simulink model "EVX_Lap_Simulation 2"  (R2018b)
settings: Solver=FixedStepAuto  StartTime=0  StopTime=120  FixedStep=0.001  MaxStep=0.01  RelTol=1e-2
values from neighbouring files (symbols this model uses):
  velocity_dnew = velocity_d + 0.4 .* (velocity_dmax - velocity_d)    [Run_Sim(with_fmincon).m]
undefined symbols (not defined in the file or in its folder): dist, theta_d
libraries: simulink x1
(part 1 of 3)
settings Model: Creator=Foster  LastModifiedBy=Foster
settings SolverCC: AlgebraicLoopSolver=LineSearch
settings DebuggingCC: UnderSpecifiedDimensionMsg=warning
settings HardwareCC: ProdBitPerLong=64  ProdHWDeviceType=Intel->x86-64 (Mac OS X)

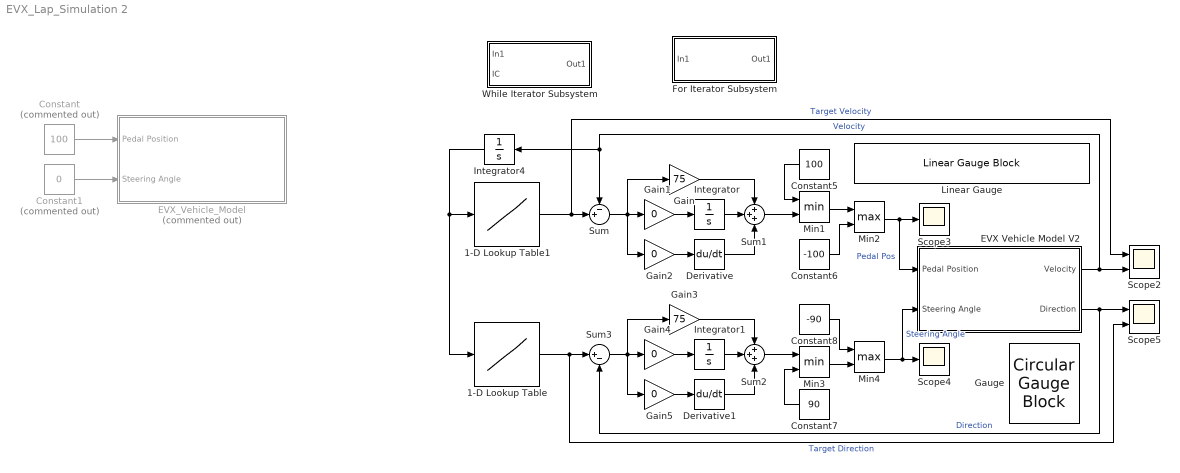
== system EVX_Lap_Simulation 2 ==
  1-D Lookup Table : Lookup_n-D  NumberOfTableDimensions=1  BreakpointsForDimension1=dist  Table=theta_d  ExtrapMethod=Clip  InternalRulePriority=Speed  RndMeth=Simplest  InputSameDT=on
  1-D Lookup Table1 : Lookup_n-D  NumberOfTableDimensions=1  BreakpointsForDimension1=dist  Table=velocity_dnew  ExtrapMethod=Clip  InternalRulePriority=Speed  RndMeth=Simplest  InputSameDT=on
  Constant : Constant  Commented=on  Value=100
  Constant1 : Constant  Commented=on  Value=0
  Constant5 : Constant  Value=100
  Constant6 : Constant  Value=-100
  Constant7 : Constant  Value=90
  Constant8 : Constant  Value=-90
  Derivative : Derivative
  Derivative1 : Derivative
  EVX Vehicle Model V2 : Subsystem
  EVX_Vehicle_Model : Subsystem  Commented=on
  For Iterator Subsystem : Subsystem  TreatAsAtomicUnit=on
  Gain : Gain  Gain=75
  Gain{1..2,4..5} (4 alike) : Gain  Gain=0
  Gain3 : Gain  Gain=75
  Gauge : CircularGaugeBlock  WebBlockId=1272  ScaleMin=-90  ScaleMax=90
  Integrator : Integrator
  Integrator1 : Integrator
  Integrator4 : Integrator
  Linear Gauge : LinearGaugeBlock  WebBlockId=1271  ScaleMin=-100
  Min1 : MinMax  Inputs=2
  Min2 : MinMax  Function=max  Inputs=2
  Min3 : MinMax  Inputs=2
  Min4 : MinMax  Function=max  Inputs=2
  Scope2 : Scope  NumInputPorts=2
  Scope3 : Scope
  Scope4 : Scope
  Scope5 : Scope  NumInputPorts=2
  Sum : Sum  Inputs=-+|
  Sum1 : Sum  Inputs=+++
  Sum2 : Sum  Inputs=+++
  Sum3 : Sum  Inputs=|+-
  While Iterator Subsystem : Subsystem  TreatAsAtomicUnit=on
  wires:
  Constant/1 -> EVX_Vehicle_Model/1(Pedal Position)
  Constant1/1 -> EVX_Vehicle_Model/2(Steering Angle)
  EVX Vehicle Model V2/1(Velocity) -> Scope2/2, Integrator4/1, Sum/1  "Velocity"
  Sum/1 -> Gain2/1, Gain/1, Gain1/1
  Integrator/1 -> Sum1/2
  Sum1/1 -> Min1/2
  Derivative/1 -> Sum1/3
  Gain/1 -> Sum1/1
  Gain1/1 -> Integrator/1
  Gain2/1 -> Derivative/1
  Constant5/1 -> Min1/1
  Derivative1/1 -> Sum2/3
  Gain5/1 -> Derivative1/1
  Gain3/1 -> Sum2/1
  Gain4/1 -> Integrator1/1
  Sum3/1 -> Gain5/1, Gain3/1, Gain4/1
  Integrator1/1 -> Sum2/2
  Min2/1 -> Scope3/1, EVX Vehicle Model V2/1(Pedal Position)  "Pedal Pos"
  Min1/1 -> Min2/1
  Constant6/1 -> Min2/2
  Min4/1 -> EVX Vehicle Model V2/2(Steering Angle), Scope4/1  "Steering Angle"
  Sum2/1 -> Min3/1
  Constant7/1 -> Min3/2
  Min3/1 -> Min4/2
  Constant8/1 -> Min4/1
  EVX Vehicle Model V2/2(Direction) -> Sum3/2, Scope5/1  "Direction"
  1-D Lookup Table/1 -> Scope5/2, Sum3/1  "Target Direction"
  1-D Lookup Table1/1 -> Scope2/1, Sum/2  "Target Velocity"
  Integrator4/1 -> 1-D Lookup Table1/1, 1-D Lookup Table/1

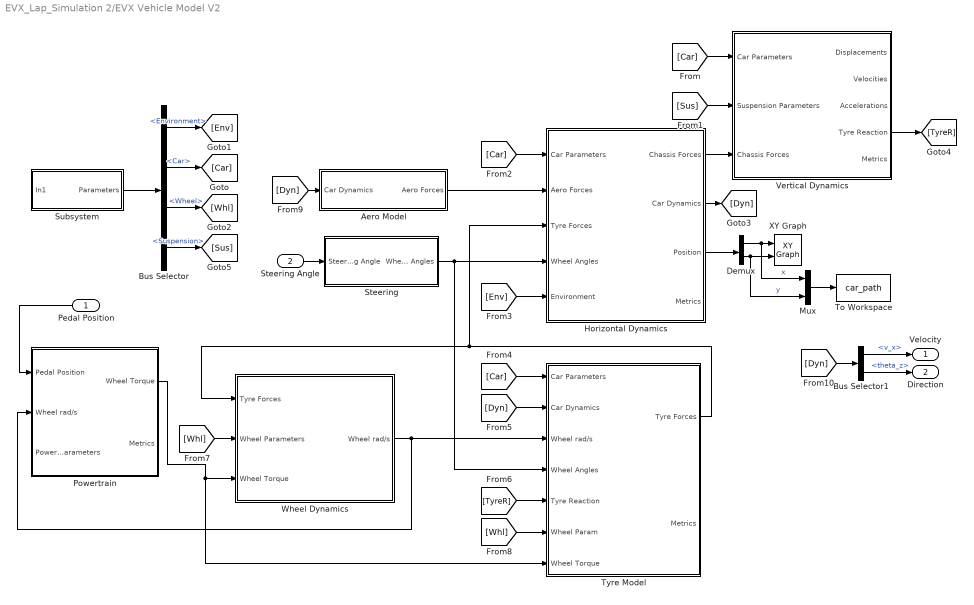
== system EVX_Lap_Simulation 2/EVX Vehicle Model V2 ==
  Pedal Position : Inport
  Steering Angle : Inport  Port=2
  Aero Model : Subsystem
  Bus Selector : BusSelector  OutputSignals=Environment,Car,Wheel,Suspension
  Bus Selector1 : BusSelector  OutputSignals=Velocities.v_x,Displacements.theta_z
  Demux : Demux  Outputs=2
  Horizontal Dynamics : Subsystem
  Mux : Mux  Inputs=2
  Powertrain : Subsystem
  Steering : Subsystem
  Subsystem : Subsystem
  To Workspace : ToWorkspace  VariableName=car_path  SaveFormat=Timeseries  SampleTime=-1
  Tyre Model : Subsystem
  Vertical Dynamics : Subsystem
  Wheel Dynamics : Subsystem
  XY Graph : simulink/Sinks/XY Graph  xmin=-400  xmax=100  ymin=-25  ymax=250  st=-1
  Velocity : Outport
  Direction : Outport  Port=2
  wires:
  [Car] -> Vertical Dynamics/1(Car Parameters)
  [Sus] -> Vertical Dynamics/2(Suspension Parameters)
  [Car] -> Horizontal Dynamics/1(Car Parameters)
  Horizontal Dynamics/3(Position) -> Demux/1
  Demux/1 -> Mux/1, XY Graph/1  "x"
  Demux/2 -> Mux/2, XY Graph/2  "y"
  Steering Angle/1 -> Steering/1(Steering Angle)
  Steering/1(Wheel Angles) -> Tyre Model/4(Wheel Angles), Horizontal Dynamics/4(Wheel Angles)
  [Env] -> Horizontal Dynamics/5(Environment)
  [Car] -> Tyre Model/1(Car Parameters)
  Horizontal Dynamics/2(Car Dynamics) -> [Dyn]
  [Dyn] -> Tyre Model/2(Car Dynamics)
  [TyreR] -> Tyre Model/5(Tyre Reaction)
  [Whl] -> Wheel Dynamics/2(Wheel Parameters)
  Pedal Position/1 -> Powertrain/1(Pedal Position)
  Powertrain/1(Wheel Torque) -> Tyre Model/7(Wheel Torque), Wheel Dynamics/3(Wheel Torque)
  [Whl] -> Tyre Model/6(Wheel Param)
  Subsystem/1(Parameters) -> Bus Selector/1
  Bus Selector/1 -> [Env]  "<Environment>"
  Bus Selector/2 -> [Car]  "<Car>"
  Bus Selector/3 -> [Whl]  "<Wheel>"
  Bus Selector/4 -> [Sus]  "<Suspension>"
  [Dyn] -> Aero Model/1(Car Dynamics)
  Aero Model/1(Aero Forces) -> Horizontal Dynamics/2(Aero Forces)
  Horizontal Dynamics/1(Chassis Forces) -> Vertical Dynamics/3(Chassis Forces)
  Vertical Dynamics/4(Tyre Reaction) -> [TyreR]
  Wheel Dynamics/1(Wheel rad/s) -> Powertrain/2(Wheel rad/s), Tyre Model/3(Wheel rad/s)
  Tyre Model/1(Tyre Forces) -> Wheel Dynamics/1(Tyre Forces), Horizontal Dynamics/3(Tyre Forces)
  [Dyn] -> Bus Selector1/1
  Bus Selector1/1 -> Velocity/1  "<v_x>"
  Bus Selector1/2 -> Direction/1  "<theta_z>"
  Mux/1 -> To Workspace/1

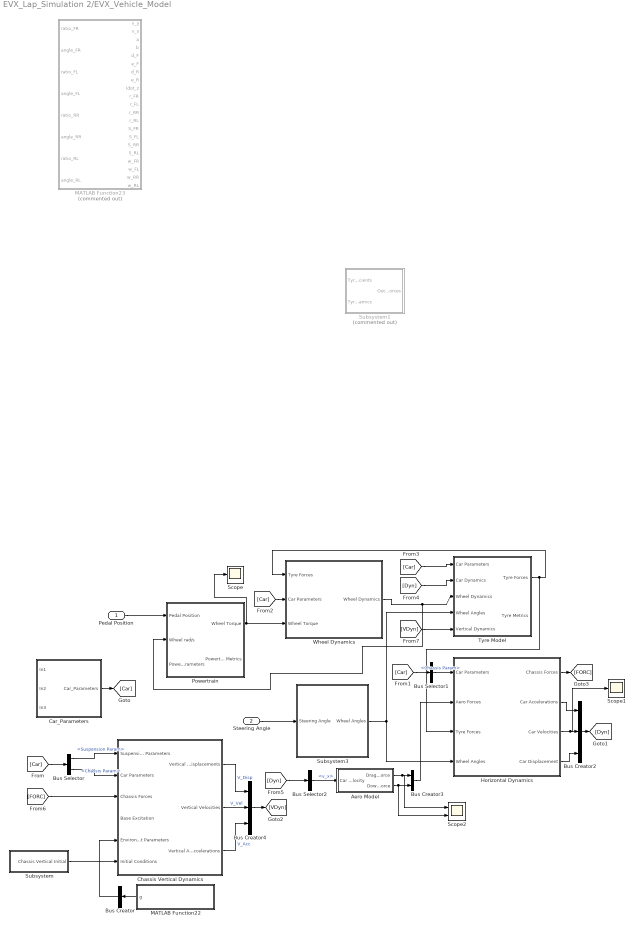
== system EVX_Lap_Simulation 2/EVX_Vehicle_Model ==
  Pedal Position : Inport
  Steering Angle : Inport  Port=2
  Aero Model : Subsystem
  Bus Creator : BusCreator  Inputs=1
  Bus Creator2 : BusCreator  Inputs=3
  Bus Creator3 : BusCreator  Inputs=2
  Bus Creator4 : BusCreator  Inputs=3
  Bus Selector : BusSelector  OutputSignals=Suspension Param,Chassis Param
  Bus Selector1 : BusSelector  OutputSignals=Chassis Param
  Bus Selector2 : BusSelector  OutputSignals=Car Velocities.v_x
  Car_Parameters : Subsystem
  Chassis Vertical Dynamics : Subsystem
  Horizontal Dynamics : Subsystem
  MATLAB Function22 : MATLAB Function  TreatAsAtomicUnit=on
  MATLAB Function23 : MATLAB Function  Commented=on  TreatAsAtomicUnit=on
  Powertrain : Subsystem
  Scope : Scope
  Scope1 : Scope
  Scope2 : Scope  NumInputPorts=2
  Subsystem : Subsystem
  Subsystem1 : Subsystem  Commented=on
  Subsystem3 : Subsystem
  Tyre Model : Subsystem
  Wheel Dynamics : Subsystem
  wires:
  Subsystem/1(Chassis Vertical Initial) -> Chassis Vertical Dynamics/6(Initial Conditions)
  MATLAB Function22/1(g) -> Bus Creator/1
  Bus Selector/1 -> Chassis Vertical Dynamics/1(Suspension Parameters)  "<Suspension Param>"
  Bus Selector1/1 -> Horizontal Dynamics/1(Car Parameters)  "<Chassis Param>"
  [Car] -> Bus Selector/1
  Bus Selector/2 -> Chassis Vertical Dynamics/2(Car Parameters)  "<Chassis Param>"
  Car_Parameters/1(Car_Parameters) -> [Car]
  [Car] -> Bus Selector1/1
  Bus Creator/1 -> Chassis Vertical Dynamics/5(Environment Parameters)
  Pedal Position/1 -> Powertrain/1(Pedal Position)
  Powertrain/1(Wheel Torque) -> Wheel Dynamics/3(Wheel Torque), Scope/1
  [Car] -> Wheel Dynamics/2(Car Parameters)
  [Car] -> Tyre Model/1(Car Parameters)
  Tyre Model/1(Tyre Forces) -> Horizontal Dynamics/3(Tyre Forces), Wheel Dynamics/1(Tyre Forces)
  Horizontal Dynamics/3(Car Velocities) -> Scope1/1, Bus Creator2/2
  Horizontal Dynamics/4(Car Displacement) -> Bus Creator2/3
  Horizontal Dynamics/2(Car Accelerations) -> Bus Creator2/1
  Bus Creator2/1 -> [Dyn]
  [Dyn] -> Tyre Model/2(Car Dynamics)
  Wheel Dynamics/1(Wheel Dynamics) -> Tyre Model/3(Wheel Dynamics), Powertrain/2(Wheel rad/s)
  Subsystem3/1(Wheel Angles) -> Tyre Model/4(Wheel Angles), Horizontal Dynamics/4(Wheel Angles)
  Steering Angle/1 -> Subsystem3/1(Steering Angle)
  [Dyn] -> Bus Selector2/1
  Bus Selector2/1 -> Aero Model/1(Car Velocity)  "<v_x>"
  Aero Model/1(Drag Force) -> Scope2/1, Bus Creator3/1
  Aero Model/2(Down Force) -> Scope2/2, Bus Creator3/2
  Bus Creator3/1 -> Horizontal Dynamics/2(Aero Forces)
  Chassis Vertical Dynamics/2(Vertical Velocities) -> Bus Creator4/2  "V_Vel"
  Chassis Vertical Dynamics/1(Vertical Displacements) -> Bus Creator4/1  "V_Disp"
  Chassis Vertical Dynamics/3(Vertical Accelerations) -> Bus Creator4/3  "V_Acc"
  Bus Creator4/1 -> [VDyn]
  Horizontal Dynamics/1(Chassis Forces) -> [FORC]
  [FORC] -> Chassis Vertical Dynamics/3(Chassis Forces)
  [VDyn] -> Tyre Model/5(Vertical Dynamics)

== system EVX_Lap_Simulation 2/For Iterator Subsystem ==
  In1 : Inport
  For Iterator : ForIterator
  Out1 : Outport
  wires:
  In1/1 -> Out1/1

== system EVX_Lap_Simulation 2/While Iterator Subsystem ==
  In1 : Inport
  IC : Inport  Port=2
  While Iterator : WhileIterator  ShowIterationPort=on
  Out1 : Outport
  wires:
  IC/1 -> While Iterator/2
  In1/1 -> Out1/1

== system EVX_Lap_Simulation 2/EVX Vehicle Model V2/Aero Model ==
  Car Dynamics : Inport
  Bus Creator : BusCreator  Inputs=2
  Bus Creator1 : BusCreator  Inputs=2
  Bus Creator2 : BusCreator  Inputs=2
  Bus Selector : BusSelector  OutputSignals=Velocities.v_x
  Forces : MATLAB Function  TreatAsAtomicUnit=on
  Interpreted MATLAB Function : MATLABFcn  MATLABFcn=Vel_update  Output1D=off
  Position : MATLAB Function  TreatAsAtomicUnit=on
  Aero Forces : Outport
  wires:
  Car Dynamics/1 -> Bus Selector/1
  Bus Selector/1 -> Forces/1(v_x), Position/1(v_x)  "<v_x>"
  Forces/1(F_L) -> Bus Creator/1
  Forces/2(F_D) -> Bus Creator/2
  Position/1(L) -> Bus Creator1/1
  Position/2(D) -> Bus Creator1/2
  Bus Creator/1 -> Bus Creator2/1  "Forces"
  Bus Creator1/1 -> Bus Creator2/2  "Position"
  Bus Creator2/1 -> Aero Forces/1

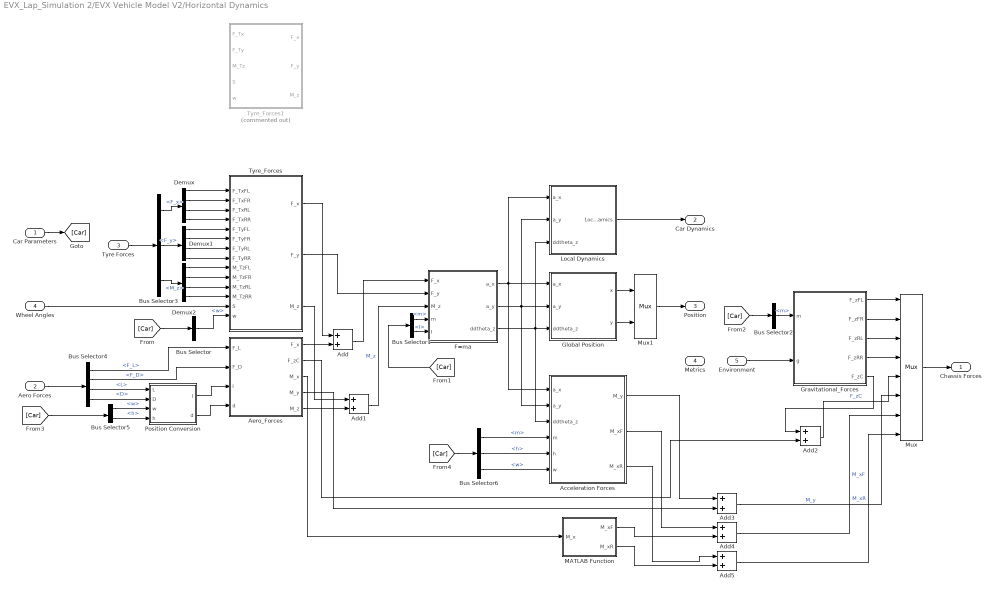
== system EVX_Lap_Simulation 2/EVX Vehicle Model V2/Horizontal Dynamics ==
  Car Parameters : Inport
  Aero Forces : Inport  Port=2
  Tyre Forces : Inport  Port=3
  Wheel Angles : Inport  Port=4
  Environment : Inport  Port=5
  Acceleration Forces : MATLAB Function  TreatAsAtomicUnit=on
  Add{,1..5} (6 alike) : Sum
  Aero_Forces : MATLAB Function  TreatAsAtomicUnit=on
  Bus Selector : BusSelector  OutputSignals=w
  Bus Selector1 : BusSelector  OutputSignals=m,I
  Bus Selector2 : BusSelector  OutputSignals=m
  Bus Selector3 : BusSelector  OutputSignals=F_x,F_y,M_z
  Bus Selector4 : BusSelector  OutputSignals=Forces.F_L,Forces.F_D,Position.L,Position.D
  Bus Selector5 : BusSelector  OutputSignals=w,h
  Bus Selector6 : BusSelector  OutputSignals=m,h,w
  Demux : Demux
  Demux1 : Demux
  Demux2 : Demux
  F=ma : MATLAB Function  TreatAsAtomicUnit=on
  Global Position : Subsystem
  Gravitational_Forces : MATLAB Function  TreatAsAtomicUnit=on
  Local Dynamics : Subsystem
  MATLAB Function : MATLAB Function  TreatAsAtomicUnit=on
  Mux : Mux  Inputs=8
      settings: DisplayOption=signals
  Mux1 : Mux  Inputs=2
      settings: DisplayOption=signals
  Position Conversion : MATLAB Function  TreatAsAtomicUnit=on
  Tyre_Forces : MATLAB Function  TreatAsAtomicUnit=on
  Tyre_Forces1 : MATLAB Function  Commented=on  TreatAsAtomicUnit=on
  Chassis Forces : Outport
  Car Dynamics : Outport  Port=2
  Position : Outport  Port=3
  Metrics : Outport  Port=4
  wires:
  Car Parameters/1 -> [Car]
  [Car] -> Bus Selector/1
  Bus Selector/1 -> Tyre_Forces/14(w)  "<w>"
  Add2/1 -> Mux/5  "F_zC"
  Add1/1 -> F=ma/3(M_z)  "M_z"
  Add/1 -> F=ma/1(F_x)
  [Car] -> Bus Selector1/1
  Bus Selector1/1 -> F=ma/4(m)  "<m>"
  Bus Selector1/2 -> F=ma/5(I)  "<I>"
  F=ma/1(a_x) -> Local Dynamics/1(a_x), Global Position/1(a_x), Acceleration Forces/1(a_x)
  F=ma/2(a_y) -> Local Dynamics/2(a_y), Global Position/2(a_y), Acceleration Forces/2(a_y)
  F=ma/3(ddtheta_z) -> Local Dynamics/3(ddtheta_z), Global Position/3(ddtheta_z), Acceleration Forces/3(ddtheta_z)
  Bus Selector2/1 -> Gravitational_Forces/1(m)  "<m>"
  [Car] -> Bus Selector2/1
  Global Position/1(x) -> Mux1/1
  Global Position/2(y) -> Mux1/2
  Mux1/1 -> Position/1
  Environment/1 -> Gravitational_Forces/2(g)
  Local Dynamics/1(Local Dynamics) -> Car Dynamics/1
  Wheel Angles/1 -> Tyre_Forces/13(S)
  Aero Forces/1 -> Bus Selector4/1
  Bus Selector4/1 -> Aero_Forces/1(F_L)  "<F_L>"
  Bus Selector4/2 -> Aero_Forces/2(F_D)  "<F_D>"
  Bus Selector4/3 -> Position Conversion/1(L)  "<L>"
  Bus Selector4/4 -> Position Conversion/2(D)  "<D>"
  Position Conversion/1(l) -> Aero_Forces/3(l)
  Position Conversion/2(d) -> Aero_Forces/4(d)
  [Car] -> Bus Selector5/1
  Bus Selector5/1 -> Position Conversion/3(w)  "<w>"
  Bus Selector5/2 -> Position Conversion/4(h)  "<h>"
  Mux/1 -> Chassis Forces/1
  [Car] -> Bus Selector6/1
  Bus Selector6/1 -> Acceleration Forces/4(m)  "<m>"
  Bus Selector6/2 -> Acceleration Forces/5(h)  "<h>"
  Bus Selector6/3 -> Acceleration Forces/6(w)  "<w>"
  Gravitational_Forces/5(F_zC) -> Add2/1
  Gravitational_Forces/4(F_zRR) -> Mux/4
  Gravitational_Forces/3(F_zRL) -> Mux/3
  Gravitational_Forces/2(F_zFR) -> Mux/2
  Gravitational_Forces/1(F_zFL) -> Mux/1
  Aero_Forces/2(F_zC) -> Add2/2
  Aero_Forces/5(M_z) -> Add1/2
  Tyre_Forces/3(M_z) -> Add1/1
  Aero_Forces/1(F_x) -> Add/2
  Tyre_Forces/1(F_x) -> Add/1
  Tyre_Forces/2(F_y) -> F=ma/2(F_y)
  Aero_Forces/3(M_x) -> MATLAB Function/1(M_x)
  Aero_Forces/4(M_y) -> Add3/2
  Acceleration Forces/1(M_y) -> Add3/1
  Add3/1 -> Mux/6  "M_y"
  Acceleration Forces/2(M_xF) -> Add4/1
  MATLAB Function/1(M_xF) -> Add4/2
  Acceleration Forces/3(M_xR) -> Add5/1
  MATLAB Function/2(M_xR) -> Add5/2
  Add4/1 -> Mux/7  "M_xF"
  Add5/1 -> Mux/8  "M_xR"
  Tyre Forces/1 -> Bus Selector3/1
  Bus Selector3/1 -> Demux/1  "<F_x>"
  Bus Selector3/2 -> Demux1/1  "<F_y>"
  Bus Selector3/3 -> Demux2/1  "<M_z>"
  Demux/1 -> Tyre_Forces/1(F_TxFL)
  Demux/2 -> Tyre_Forces/2(F_TxFR)
  Demux/3 -> Tyre_Forces/3(F_TxRL)
  Demux/4 -> Tyre_Forces/4(F_TxRR)
  Demux1/1 -> Tyre_Forces/5(F_TyFL)
  Demux1/2 -> Tyre_Forces/6(F_TyFR)
  Demux1/3 -> Tyre_Forces/7(F_TyRL)
  Demux1/4 -> Tyre_Forces/8(F_TyRR)
  Demux2/1 -> Tyre_Forces/9(M_TzFL)
  Demux2/2 -> Tyre_Forces/10(M_TzFR)
  Demux2/3 -> Tyre_Forces/11(M_TzRL)
  Demux2/4 -> Tyre_Forces/12(M_TzRR)

== system EVX_Lap_Simulation 2/EVX Vehicle Model V2/Powertrain ==
  Pedal Position : Inport
  Wheel rad/s : Inport  Port=2
  Powertrain Parameters : Inport  Port=3
  Brake Function : MATLAB Function  TreatAsAtomicUnit=on
  Constant : Constant  Value=3
  Constant1 : Constant
  Constant2 : Constant
  Demux1 : Demux
  Demux2 : Demux
  Motor Fucntion : MATLAB Function  TreatAsAtomicUnit=on
  Mux : Mux
      settings: DisplayOption=signals
  Reverse Transmission Function : MATLAB Function  TreatAsAtomicUnit=on
  Scope1 : Scope  NumInputPorts=4
  Scope2 : Scope  NumInputPorts=4
  Switch : Switch
  Transmission Function : MATLAB Function  TreatAsAtomicUnit=on
  Wheel Torque : Outport
  Metrics : Outport  Port=2
  wires:
  Constant/1 -> Transmission Function/1(Ratio), Reverse Transmission Function/1(Ratio)
  Constant1/1 -> Transmission Function/3(Splits)
  Reverse Transmission Function/1(Motor_Speed) -> Motor Fucntion/2(Motor_Speed)
  Mux/1 -> Switch/1
  Motor Fucntion/1(Torque) -> Transmission Function/2(Motor_Torque)
  Constant2/1 -> Motor Fucntion/3(Direction)
  Transmission Function/1(T_FL) -> Mux/1
  Transmission Function/2(T_FR) -> Mux/2
  Transmission Function/3(T_RL) -> Mux/3
  Transmission Function/4(T_RR) -> Mux/4
  Wheel rad/s/1 -> Demux2/1, Brake Function/1(v_wx), Reverse Transmission Function/2(dwheel)
  Demux1/4 -> Scope2/4  "T_RR"
  Demux1/3 -> Scope2/3  "T_RL"
  Demux1/1 -> Scope2/1  "T_FL"
  Demux1/2 -> Scope2/2  "T_FR"
  Pedal Position/1 -> Switch/2, Brake Function/2(Pedal), Motor Fucntion/1(Pedal)
  Switch/1 -> Demux1/1, Wheel Torque/1
  Brake Function/1(Torque) -> Switch/3
  Demux2/2 -> Scope1/2  "v_xwFR"
  Demux2/1 -> Scope1/1  "v_xwFL"
  Demux2/4 -> Scope1/4  "v_xwRR"
  Demux2/3 -> Scope1/3  "v_xwRL"

== system EVX_Lap_Simulation 2/EVX Vehicle Model V2/Steering ==
  Steering Angle : Inport
  Constant : Constant  Value=2
  Constant1 : Constant  Value=1.5
  Front/Rear Split : MATLAB Function  TreatAsAtomicUnit=on
  MATLAB Function : MATLAB Function  TreatAsAtomicUnit=on
  MATLAB Function1 : MATLAB Function  TreatAsAtomicUnit=on
  Mux : Mux
  Wheel Angles : Outport
  wires:
  Steering Angle/1 -> Front/Rear Split/1(Angle)
  Front/Rear Split/1(Steering_F) -> MATLAB Function/1(Steering_F)
  Front/Rear Split/2(Steering_R) -> MATLAB Function1/1(Steering_R)
  Constant/1 -> MATLAB Function/2(Ratio)
  Constant1/1 -> MATLAB Function1/2(Ratio)
  Mux/1 -> Wheel Angles/1
  MATLAB Function/1(S_FL) -> Mux/1
  MATLAB Function/2(S_FR) -> Mux/2
  MATLAB Function1/1(S_RL) -> Mux/3
  MATLAB Function1/2(S_RR) -> Mux/4

== system EVX_Lap_Simulation 2/EVX Vehicle Model V2/Subsystem ==
  In1 : Inport
  Bus Creator : BusCreator  Inputs=6
  Bus Creator1 : BusCreator  Inputs=6
  Bus Creator2 : BusCreator  Inputs=2
  Bus Creator3 : BusCreator  Inputs=1
  Bus Creator4 : BusCreator  Inputs=4
  Car Parameters : MATLAB Function  TreatAsAtomicUnit=on
  Environment Parameters : MATLAB Function  TreatAsAtomicUnit=on
  Suspension Parameters : MATLAB Function  TreatAsAtomicUnit=on
  Wheel Parameters : MATLAB Function  TreatAsAtomicUnit=on
  Parameters : Outport
  wires:
  Suspension Parameters/4(ct) -> Bus Creator/4
  Suspension Parameters/5(cs) -> Bus Creator/5
  Suspension Parameters/1(kt) -> Bus Creator/1
  Suspension Parameters/3(kr) -> Bus Creator/3
  Bus Creator/1 -> Bus Creator4/4  "Suspension"
  Car Parameters/1(w) -> Bus Creator1/1
  Bus Creator2/1 -> Bus Creator4/3  "Wheel"
  Bus Creator1/1 -> Bus Creator4/2  "Car"
  Suspension Parameters/2(ks) -> Bus Creator/2
  Car Parameters/5(cc) -> Bus Creator1/5
  Wheel Parameters/2(I) -> Bus Creator2/2
  Car Parameters/3(I) -> Bus Creator1/3
  Suspension Parameters/6(cr) -> Bus Creator/6
  Car Parameters/2(m) -> Bus Creator1/2
  Car Parameters/4(kc) -> Bus Creator1/4
  Wheel Parameters/1(r) -> Bus Creator2/1
  Environment Parameters/1(g) -> Bus Creator3/1
  Bus Creator3/1 -> Bus Creator4/1  "Environment"
  Bus Creator4/1 -> Parameters/1
  Car Parameters/6(h) -> Bus Creator1/6

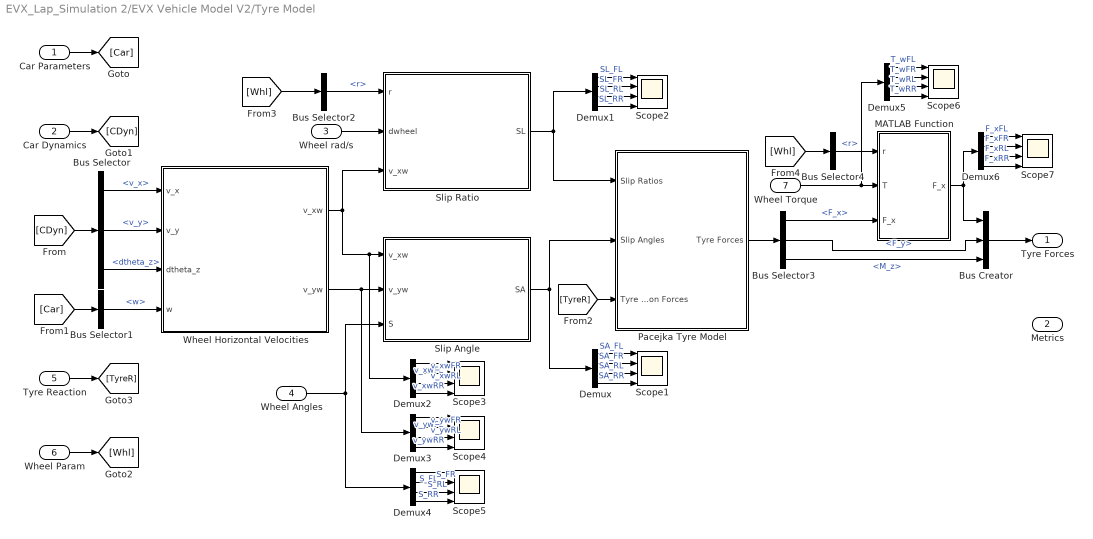
== system EVX_Lap_Simulation 2/EVX Vehicle Model V2/Tyre Model ==
  Car Parameters : Inport
  Car Dynamics : Inport  Port=2
  Wheel rad/s : Inport  Port=3
  Wheel Angles : Inport  Port=4
  Tyre Reaction : Inport  Port=5
  Wheel Param : Inport  Port=6
  Wheel Torque : Inport  Port=7
  Bus Creator : BusCreator  Inputs=3
  Bus Selector : BusSelector  OutputSignals=Velocities.v_x,Velocities.v_y,Velocities.dtheta_z
  Bus Selector1 : BusSelector  OutputSignals=w
  Bus Selector2 : BusSelector  OutputSignals=r
  Bus Selector3 : BusSelector  OutputSignals=F_x,F_y,M_z
  Bus Selector4 : BusSelector  OutputSignals=r
  Demux{,1..6} (7 alike) : Demux
  MATLAB Function : MATLAB Function  TreatAsAtomicUnit=on
  Pacejka Tyre Model : Subsystem
  Scope{1..7} (7 alike) : Scope  NumInputPorts=4
  Slip Angle : MATLAB Function  TreatAsAtomicUnit=on
  Slip Ratio : MATLAB Function  TreatAsAtomicUnit=on
  Wheel Horizontal Velocities : MATLAB Function  TreatAsAtomicUnit=on
  Tyre Forces : Outport
  Metrics : Outport  Port=2
  wires:
  Car Parameters/1 -> [Car]
  Car Dynamics/1 -> [CDyn]
  Wheel rad/s/1 -> Slip Ratio/2(dwheel)
  [CDyn] -> Bus Selector/1
  Bus Selector/3 -> Wheel Horizontal Velocities/3(dtheta_z)  "<dtheta_z>"
  [Car] -> Bus Selector1/1
  Bus Selector1/1 -> Wheel Horizontal Velocities/4(w)  "<w>"
  Tyre Reaction/1 -> [TyreR]
  [TyreR] -> Pacejka Tyre Model/3(Tyre Reaction Forces)
  Slip Angle/1(SA) -> Demux/1, Pacejka Tyre Model/2(Slip Angles)
  Slip Ratio/1(SL) -> Demux1/1, Pacejka Tyre Model/1(Slip Ratios)
  Bus Selector/1 -> Wheel Horizontal Velocities/1(v_x)  "<v_x>"
  Bus Selector/2 -> Wheel Horizontal Velocities/2(v_y)  "<v_y>"
  Wheel Horizontal Velocities/1(v_xw) -> Slip Ratio/3(v_xw), Demux2/1, Slip Angle/1(v_xw)
  Wheel Horizontal Velocities/2(v_yw) -> Demux3/1, Slip Angle/2(v_yw)
  Wheel Angles/1 -> Slip Angle/3(S), Demux4/1
  Wheel Param/1 -> [Whl]
  [Whl] -> Bus Selector2/1
  Bus Selector2/1 -> Slip Ratio/1(r)  "<r>"
  Demux/1 -> Scope1/1  "SA_FL"
  Demux/2 -> Scope1/2  "SA_FR"
  Demux/3 -> Scope1/3  "SA_RL"
  Demux/4 -> Scope1/4  "SA_RR"
  Demux1/1 -> Scope2/1  "SL_FL"
  Demux1/2 -> Scope2/2  "SL_FR"
  Demux1/3 -> Scope2/3  "SL_RL"
  Demux1/4 -> Scope2/4  "SL_RR"
  Pacejka Tyre Model/1(Tyre Forces) -> Bus Selector3/1
  [Whl] -> Bus Selector4/1
  Bus Selector4/1 -> MATLAB Function/1(r)  "<r>"
  Wheel Torque/1 -> MATLAB Function/2(T), Demux5/1
  Bus Selector3/1 -> MATLAB Function/3("F_x ")  "<F_x>"
  MATLAB Function/1(F_x) -> Bus Creator/1, Demux6/1
  Bus Selector3/2 -> Bus Creator/2  "<F_y>"
  Bus Selector3/3 -> Bus Creator/3  "<M_z>"
  Bus Creator/1 -> Tyre Forces/1
  Demux2/4 -> Scope3/4  "v_xwRR"
  Demux2/1 -> Scope3/1  "v_xwFL"
  Demux2/3 -> Scope3/3  "v_xwRL"
  Demux2/2 -> Scope3/2  "v_xwFR"
  Demux3/4 -> Scope4/4  "v_ywRR"
  Demux3/1 -> Scope4/1  "v_ywFL"
  Demux3/3 -> Scope4/3  "v_ywRL"
  Demux3/2 -> Scope4/2  "v_ywFR"
  Demux4/4 -> Scope5/4  "S_RR"
  Demux4/1 -> Scope5/1  "S_FL"
  Demux4/3 -> Scope5/3  "S_RL"
  Demux4/2 -> Scope5/2  "S_FR"
  Demux5/3 -> Scope6/3  "T_wRL"
  Demux5/4 -> Scope6/4  "T_wRR"
  Demux5/1 -> Scope6/1  "T_wFL"
  Demux5/2 -> Scope6/2  "T_wFR"
  Demux6/3 -> Scope7/3  "F_xRL"
  Demux6/4 -> Scope7/4  "F_xRR"
  Demux6/1 -> Scope7/1  "F_xFL"
  Demux6/2 -> Scope7/2  "F_xFR"

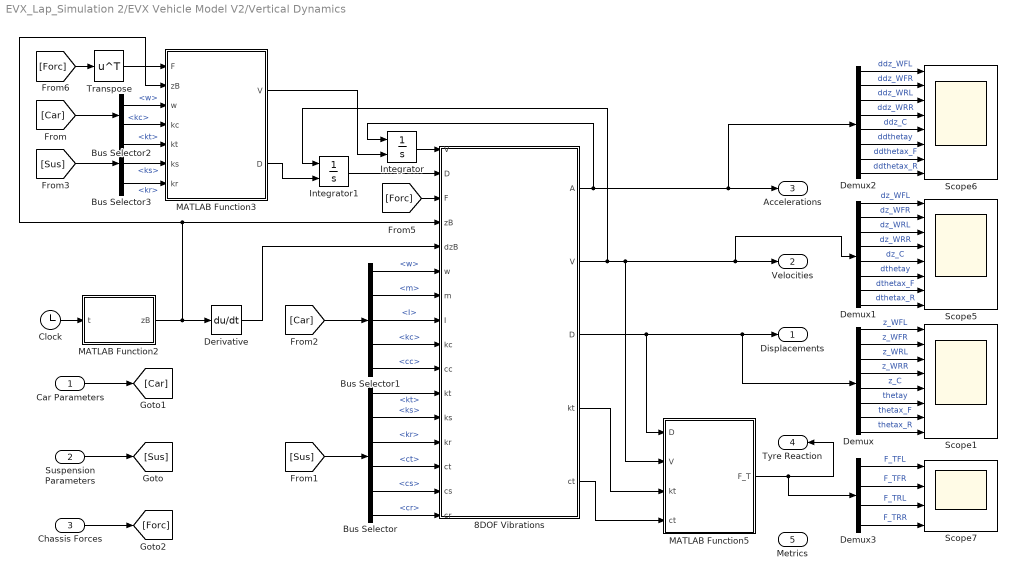
== system EVX_Lap_Simulation 2/EVX Vehicle Model V2/Vertical Dynamics ==
  Car Parameters : Inport
  Suspension Parameters : Inport  Port=2
  Chassis Forces : Inport  Port=3
  8DOF Vibrations : MATLAB Function  TreatAsAtomicUnit=on
  Bus Selector : BusSelector  OutputSignals=kt,ks,kr,ct,cs,cr
  Bus Selector1 : BusSelector  OutputSignals=w,m,I,kc,cc
  Bus Selector2 : BusSelector  OutputSignals=w,kc
  Bus Selector3 : BusSelector  OutputSignals=kt,ks,kr
  Clock : Clock
  Demux : Demux  Outputs=8
  Demux1 : Demux  Outputs=8
  Demux2 : Demux  Outputs=8
  Demux3 : Demux
  Derivative : Derivative
  Integrator : Integrator  InitialConditionSource=external
  Integrator1 : Integrator  InitialConditionSource=external
  MATLAB Function2 : MATLAB Function  TreatAsAtomicUnit=on
  MATLAB Function3 : MATLAB Function  TreatAsAtomicUnit=on
  MATLAB Function5 : MATLAB Function  TreatAsAtomicUnit=on
  Scope1 : Scope  NumInputPorts=8
  Scope5 : Scope  NumInputPorts=8
  Scope6 : Scope  NumInputPorts=8
  Scope7 : Scope  NumInputPorts=4
  Transpose : Math  Operator=transpose  SaturateOnIntegerOverflow=on
  Displacements : Outport
  Velocities : Outport  Port=2
  Accelerations : Outport  Port=3
  Tyre Reaction : Outport  Port=4
  Metrics : Outport  Port=5
  wires:
  Demux/1 -> Scope1/1  "z_WFL"
  Demux/2 -> Scope1/2  "z_WFR"
  Demux/3 -> Scope1/3  "z_WRL"
  Demux/4 -> Scope1/4  "z_WRR"
  Demux/5 -> Scope1/5  "z_C"
  Demux/6 -> Scope1/6  "thetay"
  Demux/7 -> Scope1/7  "thetax_F"
  Demux/8 -> Scope1/8  "thetax_R"
  8DOF Vibrations/3(D) -> Displacements/1, Demux/1, MATLAB Function5/1(D)
  Demux1/1 -> Scope5/1  "dz_WFL"
  Demux1/3 -> Scope5/3  "dz_WRL"
  Demux1/2 -> Scope5/2  "dz_WFR"
  Demux1/4 -> Scope5/4  "dz_WRR"
  Demux1/8 -> Scope5/8  "dthetax_R"
  Demux1/6 -> Scope5/6  "dthetay"
  Demux1/5 -> Scope5/5  "dz_C"
  Demux1/7 -> Scope5/7  "dthetax_F"
  8DOF Vibrations/2(V) -> Velocities/1, Demux1/1, MATLAB Function5/2(V), Integrator1/1
  Demux2/1 -> Scope6/1  "ddz_WFL"
  Demux2/3 -> Scope6/3  "ddz_WRL"
  Demux2/2 -> Scope6/2  "ddz_WFR"
  Demux2/4 -> Scope6/4  "ddz_WRR"
  Demux2/8 -> Scope6/8  "ddthetax_R"
  Demux2/6 -> Scope6/6  "ddthetay"
  Demux2/5 -> Scope6/5  "ddz_C"
  Demux2/7 -> Scope6/7  "ddthetax_F"
  8DOF Vibrations/1(A) -> Integrator/1, Accelerations/1, Demux2/1
  Demux3/1 -> Scope7/1  "F_TFL"
  Demux3/3 -> Scope7/3  "F_TRL"
  Demux3/2 -> Scope7/2  "F_TFR"
  Demux3/4 -> Scope7/4  "F_TRR"
  8DOF Vibrations/4(kt) -> MATLAB Function5/3(kt)
  8DOF Vibrations/5(ct) -> MATLAB Function5/4(ct)
  MATLAB Function2/1(zB) -> 8DOF Vibrations/4(zB), MATLAB Function3/2(zB), Derivative/1
  Derivative/1 -> 8DOF Vibrations/5(dzB)
  Integrator1/1 -> 8DOF Vibrations/2("D ")
  Integrator/1 -> 8DOF Vibrations/1("V ")
  Clock/1 -> MATLAB Function2/1(t)
  Suspension Parameters/1 -> [Sus]
  Car Parameters/1 -> [Car]
  [Sus] -> Bus Selector/1
  Bus Selector/1 -> 8DOF Vibrations/11("kt ")  "<kt>"
  Bus Selector/2 -> 8DOF Vibrations/12(ks)  "<ks>"
  Bus Selector/3 -> 8DOF Vibrations/13(kr)  "<kr>"
  Bus Selector/4 -> 8DOF Vibrations/14("ct ")  "<ct>"
  Bus Selector/5 -> 8DOF Vibrations/15(cs)  "<cs>"
  Bus Selector/6 -> 8DOF Vibrations/16(cr)  "<cr>"
  [Car] -> Bus Selector1/1
  Bus Selector1/1 -> 8DOF Vibrations/6(w)  "<w>"
  Bus Selector1/2 -> 8DOF Vibrations/7(m)  "<m>"
  Bus Selector1/4 -> 8DOF Vibrations/9(kc)  "<kc>"
  Bus Selector1/5 -> 8DOF Vibrations/10(cc)  "<cc>"
  [Car] -> Bus Selector2/1
  Bus Selector2/1 -> MATLAB Function3/3(w)  "<w>"
  Bus Selector2/2 -> MATLAB Function3/4(kc)  "<kc>"
  [Sus] -> Bus Selector3/1
  Bus Selector3/1 -> MATLAB Function3/5(kt)  "<kt>"
  Bus Selector3/2 -> MATLAB Function3/6(ks)  "<ks>"
  Bus Selector3/3 -> MATLAB Function3/7(kr)  "<kr>"
  MATLAB Function5/1(F_T) -> Demux3/1, Tyre Reaction/1
  MATLAB Function3/1(V) -> Integrator/2
  MATLAB Function3/2(D) -> Integrator1/2
  Bus Selector1/3 -> 8DOF Vibrations/8(I)  "<I>"
  Chassis Forces/1 -> [Forc]
  [Forc] -> 8DOF Vibrations/3(F)
  [Forc] -> Transpose/1
  Transpose/1 -> MATLAB Function3/1(F)

== system EVX_Lap_Simulation 2/EVX Vehicle Model V2/Wheel Dynamics ==
  Tyre Forces : Inport
  Wheel Parameters : Inport  Port=2
  Wheel Torque : Inport  Port=3
  Bus Selector : BusSelector  OutputSignals=F_x
  Bus Selector1 : BusSelector  OutputSignals=I,r
  Integrator : Integrator
  Scope{,1..3} (4 alike) : Scope
  Scope4 : Scope  NumInputPorts=2
  Wheel Acceleration : MATLAB Function  TreatAsAtomicUnit=on
  Wheel rad/s : Outport
  wires:
  Wheel Acceleration/1(ddwheel) -> Scope4/1, Integrator/1
  Wheel Parameters/1 -> Bus Selector1/1
  Bus Selector1/1 -> Scope/1, Wheel Acceleration/3(I)  "<I>"
  Bus Selector1/2 -> Scope3/1, Wheel Acceleration/4(r)  "<r>"
  Tyre Forces/1 -> Bus Selector/1
  Bus Selector/1 -> Scope2/1, Wheel Acceleration/1(F_x)  "<F_x>"
  Wheel Torque/1 -> Scope1/1, Wheel Acceleration/2(T)
  Integrator/1 -> Scope4/2, Wheel rad/s/1

== system EVX_Lap_Simulation 2/EVX_Vehicle_Model/Aero Model ==
  Car Velocity : Inport
  MATLAB Function : MATLAB Function  TreatAsAtomicUnit=on
  MATLAB Function1 : MATLAB Function  TreatAsAtomicUnit=on
  Drag Force : Outport
  Down Force : Outport  Port=2
  wires:
  MATLAB Function1/1(F_z) -> Down Force/1
  MATLAB Function/1(F_d) -> Drag Force/1
  Car Velocity/1 -> MATLAB Function1/1(v_x), MATLAB Function/1(v_x)

== system EVX_Lap_Simulation 2/EVX_Vehicle_Model/Car_Parameters ==
  In1 : Inport
  In2 : Inport  Port=2
  In3 : Inport  Port=3
  Bus Creator : BusCreator  Inputs=23
  Bus Creator1 : BusCreator  Inputs=4
  Bus Creator2 : BusCreator  Inputs=8
  Bus Creator6 : BusCreator  Inputs=59
  Bus Creator7 : BusCreator  Inputs=30
  MATLAB Function : MATLAB Function  TreatAsAtomicUnit=on
  MATLAB Function17 : MATLAB Function  TreatAsAtomicUnit=on
  MATLAB Function20 : MATLAB Function  TreatAsAtomicUnit=on
  MATLAB Function21 : MATLAB Function  TreatAsAtomicUnit=on
  Scope : Scope
  Car_Parameters : Outport
  wires:
  In1/1 -> MATLAB Function21/1(whatever)
  In2/1 -> MATLAB Function21/2(Owen)
  In3/1 -> MATLAB Function21/3(wants)
  MATLAB Function21/1(k_SFR) -> Bus Creator7/1
  MATLAB Function21/2(k_SFL) -> Bus Creator7/2
  MATLAB Function21/3(k_SRR) -> Bus Creator7/3
  MATLAB Function21/4(k_SRL) -> Bus Creator7/4
  MATLAB Function21/5(c_SFR) -> Bus Creator7/5
  MATLAB Function21/6(c_SFL) -> Bus Creator7/6
  MATLAB Function21/7(c_SRR) -> Bus Creator7/7
  MATLAB Function21/8(c_SRL) -> Bus Creator7/8
  MATLAB Function21/9(k_TFR) -> Bus Creator7/9
  MATLAB Function21/10(k_TFL) -> Bus Creator7/10
  MATLAB Function21/11(k_TRR) -> Bus Creator7/11
  MATLAB Function21/12(k_TRL) -> Bus Creator7/12
  MATLAB Function21/13(c_TFR) -> Bus Creator7/13
  MATLAB Function21/14(c_TFL) -> Bus Creator7/14
  MATLAB Function21/15(c_TRR) -> Bus Creator7/15
  MATLAB Function21/16(c_TRL) -> Bus Creator7/16
  MATLAB Function21/17(k_RF) -> Bus Creator7/17
  MATLAB Function21/18(k_RR) -> Bus Creator7/18
  MATLAB Function21/19(k_FRIC) -> Bus Creator7/19
  MATLAB Function21/20(c_RF) -> Bus Creator7/20
  MATLAB Function21/21(c_RR) -> Bus Creator7/21
  MATLAB Function21/22(c_FRIC) -> Bus Creator7/22
  MATLAB Function21/23(gamma_FR) -> Bus Creator7/23
  MATLAB Function21/24(gamma_FL) -> Bus Creator7/24
  MATLAB Function21/25(gamma_RR) -> Bus Creator7/25
  MATLAB Function21/26(gamma_RL) -> Bus Creator7/26
  MATLAB Function21/27(I_WFR) -> Bus Creator7/27
  MATLAB Function21/28(I_WFL) -> Bus Creator7/28
  MATLAB Function21/29(I_WRR) -> Bus Creator7/29
  MATLAB Function21/30(I_WRL) -> Bus Creator7/30
  MATLAB Function17/1(m_C) -> Bus Creator/1
  MATLAB Function17/2(m_CF) -> Bus Creator/2
  MATLAB Function17/3(m_CR) -> Bus Creator/3
  MATLAB Function17/4(m_WFR) -> Bus Creator/4
  MATLAB Function17/5(m_WFL) -> Bus Creator/5
  MATLAB Function17/6(m_WRR) -> Bus Creator/6
  MATLAB Function17/7(m_WRL) -> Bus Creator/7
  MATLAB Function17/8(I_Cy) -> Bus Creator/8
  MATLAB Function17/9(I_CFx) -> Bus Creator/9
  MATLAB Function17/10(I_CRx) -> Bus Creator/10
  MATLAB Function17/11(I_z) -> Bus Creator/11
  MATLAB Function17/12(a) -> Bus Creator/12
  MATLAB Function17/13(b) -> Bus Creator/13
  MATLAB Function17/14(d_F) -> Bus Creator/14
  MATLAB Function17/15(e_F) -> Bus Creator/15
  MATLAB Function17/16(d_R) -> Bus Creator/16
  MATLAB Function17/17(e_R) -> Bus Creator/17
  MATLAB Function17/18(k_C) -> Bus Creator/18
  MATLAB Function17/19(c_C) -> Bus Creator/19
  MATLAB Function17/20(h_C) -> Bus Creator/20
  MATLAB Function17/21(h_CF) -> Bus Creator/21
  MATLAB Function17/22(h_CR) -> Bus Creator/22
  MATLAB Function17/23(mu_scaling) -> Bus Creator/23
  MATLAB Function20/1(Fzo) -> Bus Creator6/1
  MATLAB Function20/59(p_Vx2) -> Bus Creator6/59
  MATLAB Function20/58(p_Vx1) -> Bus Creator6/58
  MATLAB Function20/57(p_Hx2) -> Bus Creator6/57
  MATLAB Function20/56(p_Hx1) -> Bus Creator6/56
  MATLAB Function20/55(p_Kx3) -> Bus Creator6/55
  MATLAB Function20/54(p_Kx2) -> Bus Creator6/54
  MATLAB Function20/53(p_Kx1) -> Bus Creator6/53
  MATLAB Function20/52(p_Ex4) -> Bus Creator6/52
  MATLAB Function20/51(p_Ex3) -> Bus Creator6/51
  MATLAB Function20/50(p_Ex2) -> Bus Creator6/50
  MATLAB Function20/49(p_Ex1) -> Bus Creator6/49
  MATLAB Function20/48(p_Dx2) -> Bus Creator6/48
  MATLAB Function20/47(p_Dx1) -> Bus Creator6/47
  MATLAB Function20/46(p_Cx1) -> Bus Creator6/46
  MATLAB Function20/45(p_Vy4) -> Bus Creator6/45
  MATLAB Function20/44(p_Vy3) -> Bus Creator6/44
  MATLAB Function20/43(p_Vy2) -> Bus Creator6/43
  MATLAB Function20/42(p_Vy1) -> Bus Creator6/42
  MATLAB Function20/41(p_Hy3) -> Bus Creator6/41
  MATLAB Function20/39(p_Hy1) -> Bus Creator6/39
  MATLAB Function20/40(p_Hy2) -> Bus Creator6/40
  MATLAB Function20/38(p_Ky3) -> Bus Creator6/38
  MATLAB Function20/37(p_Ky2) -> Bus Creator6/37
  MATLAB Function20/36(p_Ky1) -> Bus Creator6/36
  MATLAB Function20/35(p_Ey4) -> Bus Creator6/35
  MATLAB Function20/34(p_Ey3) -> Bus Creator6/34
  MATLAB Function20/33(p_Ey2) -> Bus Creator6/33
  MATLAB Function20/32(p_Ey1) -> Bus Creator6/32
  MATLAB Function20/31(p_Dy3) -> Bus Creator6/31
  MATLAB Function20/2(Ro) -> Bus Creator6/2
  MATLAB Function20/3(q_Bz1) -> Bus Creator6/3
  MATLAB Function20/4(q_Bz2) -> Bus Creator6/4
  MATLAB Function20/5(q_Bz3) -> Bus Creator6/5
  MATLAB Function20/6(q_Bz4) -> Bus Creator6/6
  MATLAB Function20/7(q_Bz5) -> Bus Creator6/7
  MATLAB Function20/8(q_Bz9) -> Bus Creator6/8
  MATLAB Function20/9(q_Bz10) -> Bus Creator6/9
  MATLAB Function20/10(q_Cz1) -> Bus Creator6/10
  MATLAB Function20/11(q_Dz1) -> Bus Creator6/11
  MATLAB Function20/12(q_Dz2) -> Bus Creator6/12
  MATLAB Function20/13(q_Dz3) -> Bus Creator6/13
  MATLAB Function20/14(q_Dz4) -> Bus Creator6/14
  MATLAB Function20/15(q_Dz6) -> Bus Creator6/15
  MATLAB Function20/16(q_Dz7) -> Bus Creator6/16
  MATLAB Function20/17(q_Dz8) -> Bus Creator6/17
  MATLAB Function20/18(q_Dz9) -> Bus Creator6/18
  MATLAB Function20/19(q_Ez1) -> Bus Creator6/19
  MATLAB Function20/20(q_Ez2) -> Bus Creator6/20
  MATLAB Function20/21(q_Ez3) -> Bus Creator6/21
  MATLAB Function20/22(q_Ez4) -> Bus Creator6/22
  MATLAB Function20/23(q_Ez5) -> Bus Creator6/23
  MATLAB Function20/24(q_Hz1) -> Bus Creator6/24
  MATLAB Function20/25(q_Hz2) -> Bus Creator6/25
  MATLAB Function20/26(q_Hz3) -> Bus Creator6/26
  MATLAB Function20/27(q_Hz4) -> Bus Creator6/27
  MATLAB Function20/28(p_Cy1) -> Bus Creator6/28
  MATLAB Function20/29(p_Dy1) -> Bus Creator6/29
  MATLAB Function20/30(p_Dy2) -> Bus Creator6/30
  Bus Creator7/1 -> Bus Creator1/1  "Suspension Param"
  Bus Creator/1 -> Scope/1, Bus Creator1/2  "Chassis Param"
  Bus Creator6/1 -> Bus Creator1/3  "Tyre Param"
  Bus Creator1/1 -> Car_Parameters/1
  MATLAB Function/1(r_FR) -> Bus Creator2/1
  MATLAB Function/2(r_FL) -> Bus Creator2/2
  MATLAB Function/3(r_RR) -> Bus Creator2/3
  MATLAB Function/4(r_RL) -> Bus Creator2/4
  Bus Creator2/1 -> Bus Creator1/4  "Wheel Param"
  MATLAB Function/5(I_FR) -> Bus Creator2/5
  MATLAB Function/6(I_FL) -> Bus Creator2/6
  MATLAB Function/7(I_RR) -> Bus Creator2/7
  MATLAB Function/8(I_RL) -> Bus Creator2/8

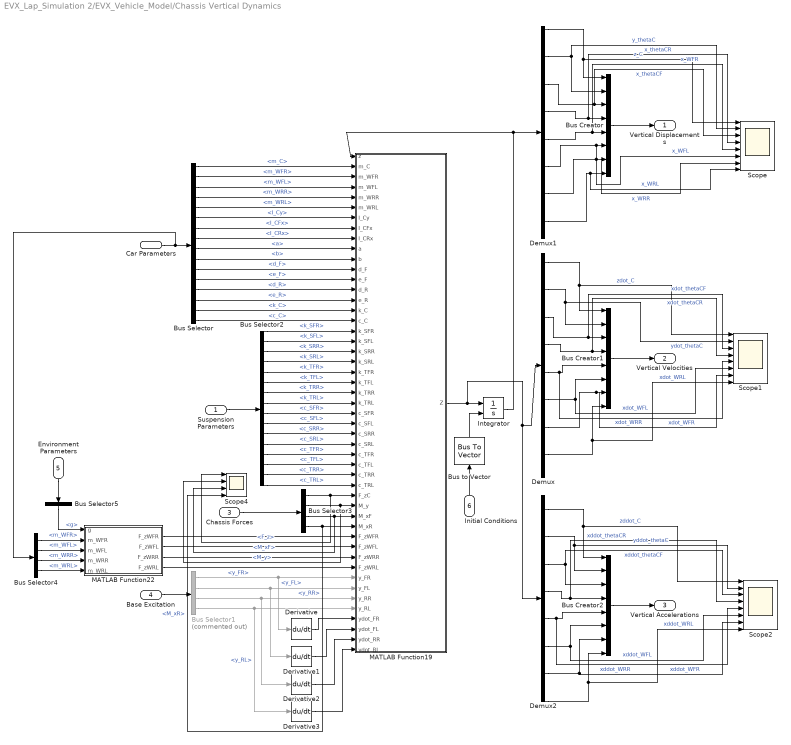
== system EVX_Lap_Simulation 2/EVX_Vehicle_Model/Chassis Vertical Dynamics ==
  Suspension Parameters : Inport
  Car Parameters : Inport  Port=2
  Chassis Forces : Inport  Port=3
  Base Excitation : Inport  Port=4
  Environment Parameters : Inport  Port=5
  Initial Conditions : Inport  Port=6
  Bus Creator : BusCreator  Inputs=8
  Bus Creator1 : BusCreator  Inputs=8
  Bus Creator2 : BusCreator  Inputs=8
  Bus Selector : BusSelector  OutputSignals=m_C,m_WFR,m_WFL,m_WRR,m_WRL,I_Cy,I_CFx,I_CRx,a,b,d_F,e_F,d_R,e_R,k_C,c_C
  Bus Selector1 : BusSelector  Commented=on  OutputSignals=y_FR,y_FL,y_RR,y_RL
  Bus Selector2 : BusSelector  OutputSignals=k_SFR,k_SFL,k_SRR,k_SRL,k_TFR,k_TFL,k_TRR,k_TRL,c_SFR,c_SFL,c_SRR,c_SRL,c_TFR,c_TFL,c_TRR,c_TRL
  Bus Selector3 : BusSelector  OutputSignals=F_z,M_y,M_xF,M_xR
  Bus Selector4 : BusSelector  OutputSignals=m_WFR,m_WFL,m_WRR,m_WRL
  Bus Selector5 : BusSelector  OutputSignals=g
  Bus to Vector : BusToVector
  Demux : Demux  Outputs=16
  Demux1 : Demux  Outputs=16
  Demux2 : Demux  Outputs=16
  Derivative{,1..3} (4 alike) : Derivative
  Integrator : Integrator  InitialConditionSource=external
  MATLAB Function19 : MATLAB Function  TreatAsAtomicUnit=on
  MATLAB Function22 : MATLAB Function  TreatAsAtomicUnit=on
  Scope : Scope  NumInputPorts=8
  Scope1 : Scope  NumInputPorts=8
  Scope2 : Scope  NumInputPorts=8
  Scope4 : Scope  NumInputPorts=4
  Vertical Displacements : Outport
  Vertical Velocities : Outport  Port=2
  Vertical Accelerations : Outport  Port=3
  wires:
  Car Parameters/1 -> Bus Selector4/1, Bus Selector/1
  Bus Selector/1 -> MATLAB Function19/2(m_C)  "<m_C>"
  Bus Selector/2 -> MATLAB Function19/3(m_WFR)  "<m_WFR>"
  Bus Selector/3 -> MATLAB Function19/4(m_WFL)  "<m_WFL>"
  Bus Selector/4 -> MATLAB Function19/5(m_WRR)  "<m_WRR>"
  Bus Selector/5 -> MATLAB Function19/6(m_WRL)  "<m_WRL>"
  Bus Selector/6 -> MATLAB Function19/7(I_Cy)  "<I_Cy>"
  Bus Selector/7 -> MATLAB Function19/8(I_CFx)  "<I_CFx>"
  Bus Selector/8 -> MATLAB Function19/9(I_CRx)  "<I_CRx>"
  Bus Selector/9 -> MATLAB Function19/10(a)  "<a>"
  MATLAB Function19/1(Z) -> Demux2/1, Demux/1, Integrator/1
  Demux1/1 -> Bus Creator/1, Scope/1  "z_C"
  Demux1/3 -> Bus Creator/2, Scope/2  "y_thetaC"
  Demux1/5 -> Scope/3, Bus Creator/3  "x_thetaCF"
  Demux1/7 -> Scope/4, Bus Creator/4  "x_thetaCR"
  Demux1/9 -> Scope/5, Bus Creator/5  "x_WFR"
  Demux1/11 -> Scope/6, Bus Creator/6  "x_WFL"
  Demux1/13 -> Scope/7, Bus Creator/7  "x_WRR"
  Demux1/15 -> Scope/8, Bus Creator/8  "x_WRL"
  Bus Creator/1 -> Vertical Displacements/1
  Bus Creator1/1 -> Vertical Velocities/1
  Bus Creator2/1 -> Vertical Accelerations/1
  Demux/1 -> Scope1/1, Bus Creator1/1  "zdot_C"
  Demux/3 -> Scope1/2, Bus Creator1/2  "ydot_thetaC"
  Demux/5 -> Scope1/3, Bus Creator1/3  "xdot_thetaCF"
  Demux/7 -> Scope1/4, Bus Creator1/4  "xdot_thetaCR"
  Demux/9 -> Scope1/5, Bus Creator1/5  "xdot_WFR"
  Demux/11 -> Bus Creator1/6, Scope1/6  "xdot_WFL"
  Demux/13 -> Scope1/7, Bus Creator1/7  "xdot_WRR"
  Demux/15 -> Scope1/8, Bus Creator1/8  "xdot_WRL"
  Demux2/2 -> Scope2/1, Bus Creator2/1  "zddot_C"
  Demux2/4 -> Bus Creator2/2, Scope2/2  "yddot_thetaC"
  Demux2/6 -> Bus Creator2/3, Scope2/3  "xddot_thetaCF"
  Demux2/8 -> Scope2/4, Bus Creator2/4  "xddot_thetaCR"
  Demux2/10 -> Scope2/5, Bus Creator2/5  "xddot_WFR"
  Demux2/12 -> Bus Creator2/6, Scope2/6  "xddot_WFL"
  Demux2/14 -> Bus Creator2/7, Scope2/7  "xddot_WRR"
  Demux2/16 -> Scope2/8, Bus Creator2/8  "xddot_WRL"
  Base Excitation/1 -> Bus Selector1/1
  Bus Selector1/1 -> Derivative/1, MATLAB Function19/42(y_FR)  "<y_FR>"
  Bus Selector1/2 -> Derivative1/1, MATLAB Function19/43(y_FL)  "<y_FL>"
  Bus Selector1/3 -> Derivative2/1, MATLAB Function19/44(y_RR)  "<y_RR>"
  Bus Selector1/4 -> Derivative3/1, MATLAB Function19/45(y_RL)  "<y_RL>"
  Derivative/1 -> MATLAB Function19/46(ydot_FR)
  Derivative1/1 -> MATLAB Function19/47(ydot_FL)
  Derivative2/1 -> MATLAB Function19/48(ydot_RR)
  Derivative3/1 -> MATLAB Function19/49(ydot_RL)
  Suspension Parameters/1 -> Bus Selector2/1
  Bus Selector2/1 -> MATLAB Function19/18(k_SFR)  "<k_SFR>"
  Bus Selector2/2 -> MATLAB Function19/19(k_SFL)  "<k_SFL>"
  Bus Selector2/3 -> MATLAB Function19/20(k_SRR)  "<k_SRR>"
  Bus Selector2/4 -> MATLAB Function19/21(k_SRL)  "<k_SRL>"
  Bus Selector2/9 -> MATLAB Function19/26(c_SFR)  "<c_SFR>"
  Bus Selector2/10 -> MATLAB Function19/27(c_SFL)  "<c_SFL>"
  Bus Selector2/11 -> MATLAB Function19/28(c_SRR)  "<c_SRR>"
  Bus Selector2/12 -> MATLAB Function19/29(c_SRL)  "<c_SRL>"
  Bus Selector2/5 -> MATLAB Function19/22(k_TFR)  "<k_TFR>"
  Bus Selector2/6 -> MATLAB Function19/23(k_TFL)  "<k_TFL>"
  Bus Selector2/7 -> MATLAB Function19/24(k_TRR)  "<k_TRR>"
  Bus Selector2/8 -> MATLAB Function19/25(k_TRL)  "<k_TRL>"
  Bus Selector2/13 -> MATLAB Function19/30(c_TFR)  "<c_TFR>"
  Bus Selector2/14 -> MATLAB Function19/31(c_TFL)  "<c_TFL>"
  Bus Selector2/15 -> MATLAB Function19/32(c_TRR)  "<c_TRR>"
  Bus Selector2/16 -> MATLAB Function19/33(c_TRL)  "<c_TRL>"
  Chassis Forces/1 -> Bus Selector3/1
  Bus Selector3/1 -> Scope4/1, MATLAB Function19/34(F_zC)  "<F_z>"
  Bus Selector3/2 -> Scope4/2, MATLAB Function19/35(M_y)  "<M_y>"
  Bus Selector3/3 -> Scope4/3, MATLAB Function19/36(M_xF)  "<M_xF>"
  Bus Selector3/4 -> MATLAB Function19/37(M_xR), Scope4/4  "<M_xR>"
  Bus Selector4/1 -> MATLAB Function22/2(m_WFR)  "<m_WFR>"
  Bus Selector4/2 -> MATLAB Function22/3(m_WFL)  "<m_WFL>"
  Bus Selector4/3 -> MATLAB Function22/4(m_WRR)  "<m_WRR>"
  Bus Selector4/4 -> MATLAB Function22/5(m_WRL)  "<m_WRL>"
  Environment Parameters/1 -> Bus Selector5/1
  MATLAB Function22/1(F_zWFR) -> MATLAB Function19/38(F_zWFR)
  MATLAB Function22/2(F_zWFL) -> MATLAB Function19/39(F_zWFL)
  MATLAB Function22/3(F_zWRR) -> MATLAB Function19/40(F_zWRR)
  MATLAB Function22/4(F_zWRL) -> MATLAB Function19/41(F_zWRL)
  Bus Selector5/1 -> MATLAB Function22/1(g)  "<g>"
  Bus Selector/10 -> MATLAB Function19/11(b)  "<b>"
  Bus Selector/11 -> MATLAB Function19/12(d_F)  "<d_F>"
  Bus Selector/12 -> MATLAB Function19/13(e_F)  "<e_F>"
  Bus Selector/13 -> MATLAB Function19/14(d_R)  "<d_R>"
  Bus Selector/14 -> MATLAB Function19/15(e_R)  "<e_R>"
  Bus Selector/15 -> MATLAB Function19/16(k_C)  "<k_C>"
  Bus Selector/16 -> MATLAB Function19/17(c_C)  "<c_C>"
  Integrator/1 -> MATLAB Function19/1(z), Demux1/1
  Initial Conditions/1 -> Bus to Vector/1
  Bus to Vector/1 -> Integrator/2

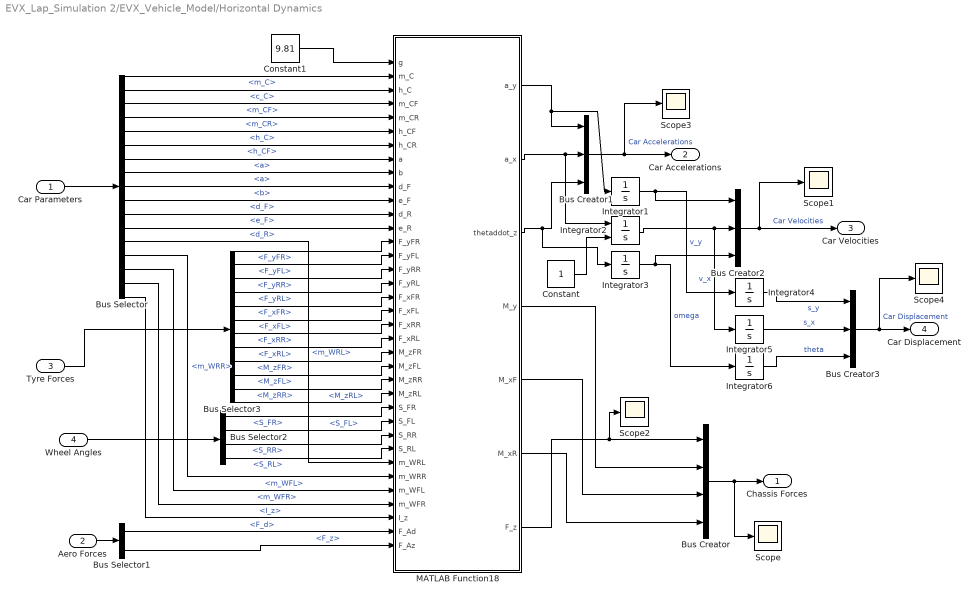
== system EVX_Lap_Simulation 2/EVX_Vehicle_Model/Horizontal Dynamics ==
  Car Parameters : Inport
  Aero Forces : Inport  Port=2
  Tyre Forces : Inport  Port=3
  Wheel Angles : Inport  Port=4
  Bus Creator : BusCreator  Inputs=4
  Bus Creator1 : BusCreator  Inputs=3
  Bus Creator2 : BusCreator  Inputs=3
  Bus Creator3 : BusCreator  Inputs=3
  Bus Selector : BusSelector  OutputSignals=m_C,c_C,m_CF,m_CR,h_C,h_CF,a,a,b,d_F,e_F,d_R,m_WRL,m_WRR,m_WFL,m_WFR,I_z
  Bus Selector1 : BusSelector  OutputSignals=F_d,F_z
  Bus Selector2 : BusSelector  OutputSignals=S_FR,S_FL,S_RR,S_RL
  Bus Selector3 : BusSelector  OutputSignals=F_y.F_yFR,F_y.F_yFL,F_y.F_yRR,F_y.F_yRL,F_x.F_xFR,F_x.F_xFL,F_x.F_xRR,F_x.F_xRL,M_z.M_zFR,M_z.M_zFL,M_z.M_zRR,M_z.M_zRL
  Constant : Constant
  Constant1 : Constant  Value=9.81
  Integrator{1,3..6} (5 alike) : Integrator
  Integrator2 : Integrator  InitialConditionSource=external
  MATLAB Function18 : MATLAB Function  TreatAsAtomicUnit=on
  Scope{,1..4} (5 alike) : Scope
  Chassis Forces : Outport
  Car Accelerations : Outport  Port=2
  Car Velocities : Outport  Port=3
  Car Displacement : Outport  Port=4
  wires:
  MATLAB Function18/7(F_z) -> Scope2/1, Bus Creator/1
  MATLAB Function18/4(M_y) -> Bus Creator/2
  MATLAB Function18/5(M_xF) -> Bus Creator/3
  MATLAB Function18/6(M_xR) -> Bus Creator/4
  Bus Creator/1 -> Scope/1, Chassis Forces/1
  Car Parameters/1 -> Bus Selector/1
  Bus Selector/1 -> MATLAB Function18/2(m_C)  "<m_C>"
  Bus Selector/2 -> MATLAB Function18/3(h_C)  "<c_C>"
  Bus Selector/3 -> MATLAB Function18/4(m_CF)  "<m_CF>"
  Bus Selector/4 -> MATLAB Function18/5(m_CR)  "<m_CR>"
  Bus Selector/5 -> MATLAB Function18/6(h_CF)  "<h_C>"
  Bus Selector/6 -> MATLAB Function18/7(h_CR)  "<h_CF>"
  Bus Selector/7 -> MATLAB Function18/8(a)  "<a>"
  Bus Selector/8 -> MATLAB Function18/9(b)  "<a>"
  Bus Selector/9 -> MATLAB Function18/10(d_F)  "<b>"
  Bus Selector/10 -> MATLAB Function18/11(e_F)  "<d_F>"
  Bus Selector/11 -> MATLAB Function18/12(d_R)  "<e_F>"
  Bus Selector/12 -> MATLAB Function18/13(e_R)  "<d_R>"
  Bus Selector/16 -> MATLAB Function18/33(m_WFR)  "<m_WFR>"
  Bus Selector/15 -> MATLAB Function18/32(m_WFL)  "<m_WFL>"
  Bus Selector/14 -> MATLAB Function18/31(m_WRR)  "<m_WRR>"
  Bus Selector/13 -> MATLAB Function18/30(m_WRL)  "<m_WRL>"
  Bus Selector/17 -> MATLAB Function18/34(I_z)  "<I_z>"
  Bus Creator1/1 -> Scope3/1, Car Accelerations/1  "Car Accelerations"
  MATLAB Function18/2(a_x) -> Integrator2/1, Bus Creator1/2
  MATLAB Function18/1(a_y) -> Integrator1/1, Bus Creator1/1
  MATLAB Function18/3(thetaddot_z) -> Integrator3/1, Bus Creator1/3
  Integrator2/1 -> Integrator5/1, Bus Creator2/2  "v_x"
  Integrator1/1 -> Bus Creator2/1, Integrator4/1  "v_y"
  Integrator3/1 -> Integrator6/1, Bus Creator2/3  "omega"
  Bus Creator2/1 -> Scope1/1, Car Velocities/1  "Car Velocities"
  Integrator4/1 -> Bus Creator3/1  "s_y"
  Integrator6/1 -> Bus Creator3/3  "theta"
  Integrator5/1 -> Bus Creator3/2  "s_x"
  Bus Creator3/1 -> Scope4/1, Car Displacement/1  "Car Displacement"
  Wheel Angles/1 -> Bus Selector2/1
  Tyre Forces/1 -> Bus Selector3/1
  Bus Selector2/1 -> MATLAB Function18/26(S_FR)  "<S_FR>"
  Bus Selector2/2 -> MATLAB Function18/27(S_FL)  "<S_FL>"
  Bus Selector2/3 -> MATLAB Function18/28(S_RR)  "<S_RR>"
  Bus Selector2/4 -> MATLAB Function18/29(S_RL)  "<S_RL>"
  Bus Selector3/1 -> MATLAB Function18/14(F_yFR)  "<F_yFR>"
  Bus Selector3/2 -> MATLAB Function18/15(F_yFL)  "<F_yFL>"
  Bus Selector3/3 -> MATLAB Function18/16(F_yRR)  "<F_yRR>"
  Bus Selector3/4 -> MATLAB Function18/17(F_yRL)  "<F_yRL>"
  Bus Selector3/5 -> MATLAB Function18/18(F_xFR)  "<F_xFR>"
  Bus Selector3/6 -> MATLAB Function18/19(F_xFL)  "<F_xFL>"
  Bus Selector3/7 -> MATLAB Function18/20(F_xRR)  "<F_xRR>"
  Bus Selector3/8 -> MATLAB Function18/21(F_xRL)  "<F_xRL>"
  Bus Selector3/9 -> MATLAB Function18/22(M_zFR)  "<M_zFR>"
  Bus Selector3/10 -> MATLAB Function18/23(M_zFL)  "<M_zFL>"
  Bus Selector3/11 -> MATLAB Function18/24(M_zRR)  "<M_zRR>"
  Bus Selector3/12 -> MATLAB Function18/25(M_zRL)  "<M_zRL>"
  Constant/1 -> Integrator2/2
  Aero Forces/1 -> Bus Selector1/1
  Bus Selector1/1 -> MATLAB Function18/35(F_Ad)  "<F_d>"
  Bus Selector1/2 -> MATLAB Function18/36(F_Az)  "<F_z>"
  Constant1/1 -> MATLAB Function18/1(g)

== system EVX_Lap_Simulation 2/EVX_Vehicle_Model/Powertrain ==
  Pedal Position : Inport
  Wheel rad/s : Inport  Port=2
  Powertrain Parameters : Inport  Port=3
  Bus Creator : BusCreator  Inputs=4
  Bus Selector : BusSelector  OutputSignals=w.w_FR,w.w_FL,w.w_RR,w.w_RL
  Constant : Constant  Value=3
  Constant1 : Constant
  Constant2 : Constant
  Motor Fucntion : MATLAB Function  TreatAsAtomicUnit=on
  Reverse Transmission Function : MATLAB Function  TreatAsAtomicUnit=on
  Scope : Scope
  Scope1 : Scope
  Transmission Function : MATLAB Function  TreatAsAtomicUnit=on
  Wheel Torque : Outport
  Powertrain Metrics : Outport  Port=2
  wires:
  Constant/1 -> Transmission Function/1(Ratio), Reverse Transmission Function/1(Ratio)
  Constant1/1 -> Transmission Function/3(Splits)
  Pedal Position/1 -> Motor Fucntion/1(Pedal)
  Reverse Transmission Function/1(Motor_Speed) -> Motor Fucntion/2(Motor_Speed)
  Transmission Function/1(T_FR) -> Bus Creator/1
  Transmission Function/2(T_FL) -> Bus Creator/2
  Transmission Function/3(T_RR) -> Bus Creator/3
  Bus Creator/1 -> Scope1/1, Wheel Torque/1
  Wheel rad/s/1 -> Bus Selector/1
  Bus Selector/1 -> Reverse Transmission Function/2(w_FR)  "<w_FR>"
  Bus Selector/2 -> Reverse Transmission Function/3(w_FL)  "<w_FL>"
  Bus Selector/3 -> Reverse Transmission Function/4(w_RR)  "<w_RR>"
  Bus Selector/4 -> Reverse Transmission Function/5(w_RL)  "<w_RL>"
  Motor Fucntion/1(Torque) -> Transmission Function/2(Motor_Torque), Scope/1
  Transmission Function/4(T_RL) -> Bus Creator/4
  Constant2/1 -> Motor Fucntion/3(Direction)

== system EVX_Lap_Simulation 2/EVX_Vehicle_Model/Subsystem ==
  Chassis Vertical Initial Conditions : MATLAB Function  TreatAsAtomicUnit=on
  Chassis Vertical Initial : Outport
  wires:
  Chassis Vertical Initial Conditions/1(Initial) -> Chassis Vertical Initial/1
